simulink model "bit4alu_subsystem"  (R2020a)
settings: Solver=VariableStepAuto  StartTime=0.0  StopTime=10.0  RelTol=1e-3
settings Model: Creator=F1  LastModifiedBy=F1

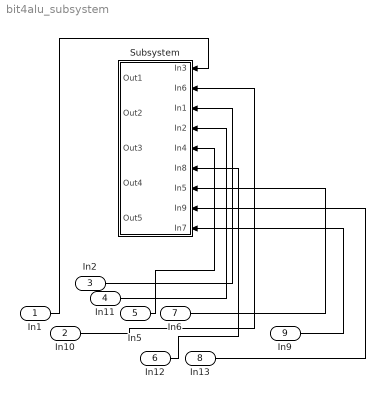
== system bit4alu_subsystem ==
  In1 : Inport
  In10 : Inport  Port=2
  In2 : Inport  Port=3
  In11 : Inport  Port=4
  In5 : Inport  Port=5
  In12 : Inport  Port=6
  In6 : Inport  Port=7
  In13 : Inport  Port=8
  In9 : Inport  Port=9
  Subsystem : Subsystem
  wires:
  In2/1 -> Subsystem/3(In1)
  In11/1 -> Subsystem/4(In2)
  In1/1 -> Subsystem/1(In3)
  In5/1 -> Subsystem/5(In4)
  In6/1 -> Subsystem/7(In5)
  In10/1 -> Subsystem/2(In6)
  In9/1 -> Subsystem/9(In7)
  In12/1 -> Subsystem/6(In8)
  In13/1 -> Subsystem/8(In9)

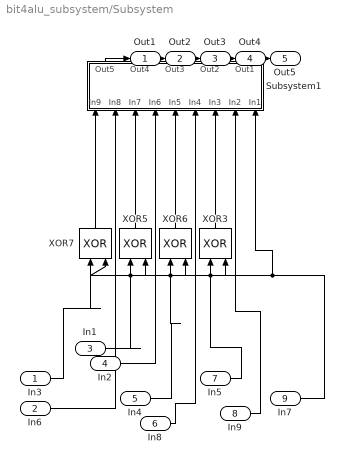
== system bit4alu_subsystem/Subsystem ==
  In3 : Inport
  In6 : Inport  Port=2
  In1 : Inport  Port=3
  In2 : Inport  Port=4
  In4 : Inport  Port=5
  In8 : Inport  Port=6
  In5 : Inport  Port=7
  In9 : Inport  Port=8
  In7 : Inport  Port=9
  Subsystem1 : Subsystem
  XOR{3,5..7} (4 alike) : Logic  Operator=XOR  IconShape=distinctive  AllPortsSameDT=off  OutDataTypeStr=boolean
  Out1 : Outport
  Out2 : Outport  Port=2
  Out3 : Outport  Port=3
  Out4 : Outport  Port=4
  Out5 : Outport  Port=5
  wires:
  XOR6/1 -> Subsystem1/5(In5)
  XOR5/1 -> Subsystem1/7(In7)
  XOR3/1 -> Subsystem1/3(In3)
  Subsystem1/1(Out1) -> Out5/1
  In7/1 -> XOR7/1, XOR5/1, XOR6/1, XOR3/1, Subsystem1/1(In1)
  Subsystem1/2(Out2) -> Out4/1
  Subsystem1/4(Out4) -> Out2/1
  Subsystem1/3(Out3) -> Out3/1
  In2/1 -> Subsystem1/6(In6)
  XOR7/1 -> Subsystem1/9(In9)
  Subsystem1/5(Out5) -> Out1/1
  In5/1 -> XOR3/2
  In1/1 -> XOR5/2
  In3/1 -> XOR7/2
  In6/1 -> Subsystem1/8(In8)
  In9/1 -> Subsystem1/2(In2)
  In4/1 -> XOR6/2
  In8/1 -> Subsystem1/4(In4)

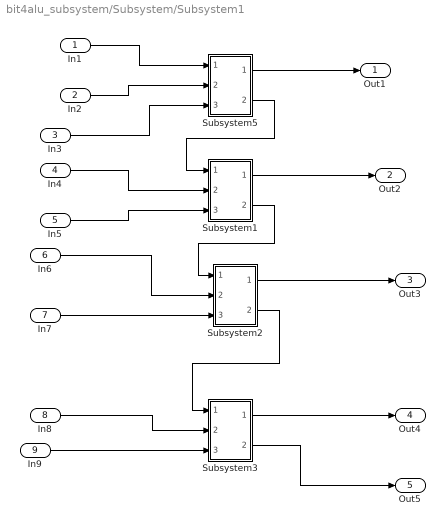
== system bit4alu_subsystem/Subsystem/Subsystem1 ==
  In1 : Inport
  In2 : Inport  Port=2
  In3 : Inport  Port=3
  In4 : Inport  Port=4
  In5 : Inport  Port=5
  In6 : Inport  Port=6
  In7 : Inport  Port=7
  In8 : Inport  Port=8
  In9 : Inport  Port=9
  Subsystem1 : Subsystem
  Subsystem2 : Subsystem
  Subsystem3 : Subsystem
  Subsystem5 : Subsystem
  Out1 : Outport
  Out2 : Outport  Port=2
  Out3 : Outport  Port=3
  Out4 : Outport  Port=4
  Out5 : Outport  Port=5
  wires:
  Subsystem2/2(Out2) -> Subsystem3/1(In1)
  In8/1 -> Subsystem3/2(In2)
  Subsystem5/2(Out2) -> Subsystem1/1(In1)
  Subsystem2/1(Out1) -> Out3/1
  Subsystem1/2(Out2) -> Subsystem2/1(In1)
  In6/1 -> Subsystem2/2(In2)
  In7/1 -> Subsystem2/3(In3)
  In4/1 -> Subsystem1/2(In2)
  Subsystem3/1(Out1) -> Out4/1
  In9/1 -> Subsystem3/3(In3)
  In2/1 -> Subsystem5/2(In2)
  In3/1 -> Subsystem5/3(In3)
  In1/1 -> Subsystem5/1(In1)
  Subsystem5/1(Out1) -> Out1/1
  Subsystem3/2(Out2) -> Out5/1
  Subsystem1/1(Out1) -> Out2/1
  In5/1 -> Subsystem1/3(In3)

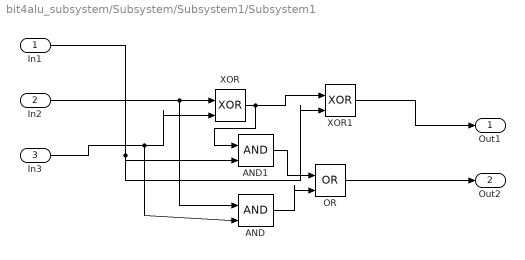
== system bit4alu_subsystem/Subsystem/Subsystem1/Subsystem1 ==
  In1 : Inport
  In2 : Inport  Port=2
  In3 : Inport  Port=3
  AND : Logic  IconShape=distinctive  AllPortsSameDT=off  OutDataTypeStr=boolean
  AND1 : Logic  IconShape=distinctive  AllPortsSameDT=off  OutDataTypeStr=boolean
  OR : Logic  Operator=OR  IconShape=distinctive  AllPortsSameDT=off  OutDataTypeStr=boolean
  XOR : Logic  Operator=XOR  IconShape=distinctive  AllPortsSameDT=off  OutDataTypeStr=boolean
  XOR1 : Logic  Operator=XOR  IconShape=distinctive  AllPortsSameDT=off  OutDataTypeStr=boolean
  Out1 : Outport
  Out2 : Outport  Port=2
  wires:
  AND1/1 -> OR/1
  AND/1 -> OR/2
  In3/1 -> AND/2, XOR/2
  In2/1 -> AND/1, XOR/1
  In1/1 -> XOR1/2, AND1/2
  XOR/1 -> AND1/1, XOR1/1
  XOR1/1 -> Out1/1
  OR/1 -> Out2/1

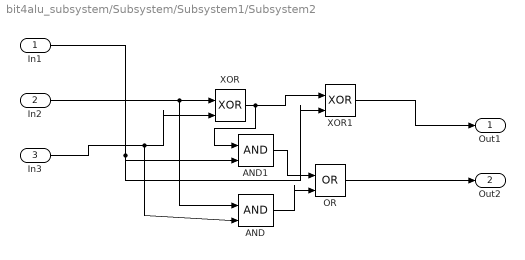
== system bit4alu_subsystem/Subsystem/Subsystem1/Subsystem2 ==
  In1 : Inport
  In2 : Inport  Port=2
  In3 : Inport  Port=3
  AND : Logic  IconShape=distinctive  AllPortsSameDT=off  OutDataTypeStr=boolean
  AND1 : Logic  IconShape=distinctive  AllPortsSameDT=off  OutDataTypeStr=boolean
  OR : Logic  Operator=OR  IconShape=distinctive  AllPortsSameDT=off  OutDataTypeStr=boolean
  XOR : Logic  Operator=XOR  IconShape=distinctive  AllPortsSameDT=off  OutDataTypeStr=boolean
  XOR1 : Logic  Operator=XOR  IconShape=distinctive  AllPortsSameDT=off  OutDataTypeStr=boolean
  Out1 : Outport
  Out2 : Outport  Port=2
  wires:
  AND1/1 -> OR/1
  AND/1 -> OR/2
  In3/1 -> AND/2, XOR/2
  In2/1 -> AND/1, XOR/1
  In1/1 -> XOR1/2, AND1/2
  XOR/1 -> AND1/1, XOR1/1
  XOR1/1 -> Out1/1
  OR/1 -> Out2/1

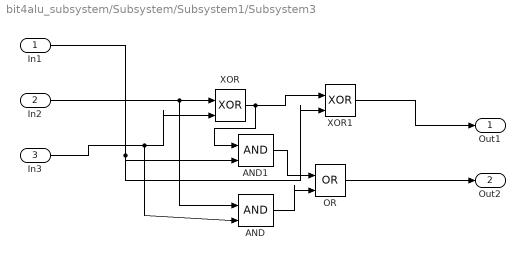
== system bit4alu_subsystem/Subsystem/Subsystem1/Subsystem3 ==
  In1 : Inport
  In2 : Inport  Port=2
  In3 : Inport  Port=3
  AND : Logic  IconShape=distinctive  AllPortsSameDT=off  OutDataTypeStr=boolean
  AND1 : Logic  IconShape=distinctive  AllPortsSameDT=off  OutDataTypeStr=boolean
  OR : Logic  Operator=OR  IconShape=distinctive  AllPortsSameDT=off  OutDataTypeStr=boolean
  XOR : Logic  Operator=XOR  IconShape=distinctive  AllPortsSameDT=off  OutDataTypeStr=boolean
  XOR1 : Logic  Operator=XOR  IconShape=distinctive  AllPortsSameDT=off  OutDataTypeStr=boolean
  Out1 : Outport
  Out2 : Outport  Port=2
  wires:
  AND1/1 -> OR/1
  AND/1 -> OR/2
  In3/1 -> AND/2, XOR/2
  In2/1 -> AND/1, XOR/1
  In1/1 -> XOR1/2, AND1/2
  XOR/1 -> AND1/1, XOR1/1
  XOR1/1 -> Out1/1
  OR/1 -> Out2/1

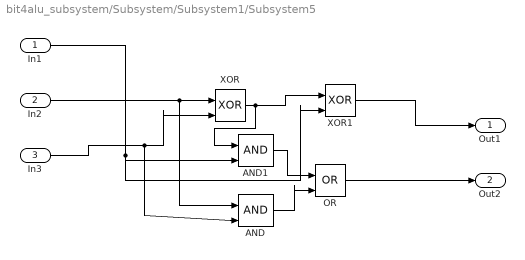
== system bit4alu_subsystem/Subsystem/Subsystem1/Subsystem5 ==
  In1 : Inport
  In2 : Inport  Port=2
  In3 : Inport  Port=3
  AND : Logic  IconShape=distinctive  AllPortsSameDT=off  OutDataTypeStr=boolean
  AND1 : Logic  IconShape=distinctive  AllPortsSameDT=off  OutDataTypeStr=boolean
  OR : Logic  Operator=OR  IconShape=distinctive  AllPortsSameDT=off  OutDataTypeStr=boolean
  XOR : Logic  Operator=XOR  IconShape=distinctive  AllPortsSameDT=off  OutDataTypeStr=boolean
  XOR1 : Logic  Operator=XOR  IconShape=distinctive  AllPortsSameDT=off  OutDataTypeStr=boolean
  Out1 : Outport
  Out2 : Outport  Port=2
  wires:
  AND1/1 -> OR/1
  AND/1 -> OR/2
  In3/1 -> AND/2, XOR/2
  In2/1 -> AND/1, XOR/1
  In1/1 -> XOR1/2, AND1/2
  XOR/1 -> AND1/1, XOR1/1
  XOR1/1 -> Out1/1
  OR/1 -> Out2/1
